simulink model "apollo_longitude"  (R2018a)
settings: Solver=VariableStepAuto  StartTime=0.0  StopTime=200  RelTol=1e-5
undefined symbols (not defined in the file): high_speed_Ki, high_speed_Kp, ref_station, speed_controller_input_limit, station_Kp
settings Model: Creator=cidi-xh  LastModifiedBy=DELL

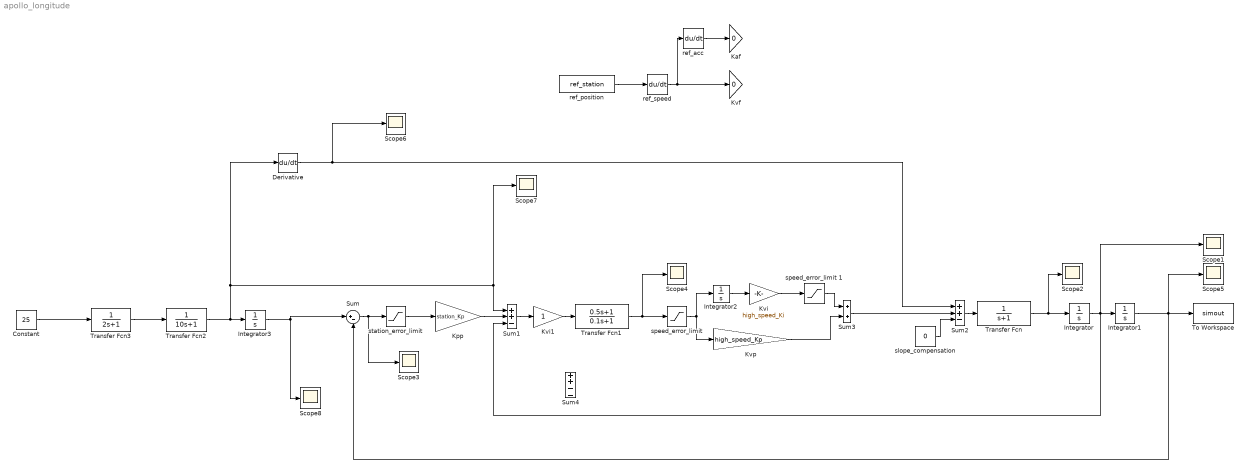
== system apollo_longitude ==
  Constant : Constant  Value=25
  Derivative : Derivative
  Integrator{,1..3} (4 alike) : Integrator
  Kaf : Gain  Gain=0
  Kpp : Gain  Gain=station_Kp
  Kvf : Gain  Gain=0
  Kvi : Gain  Gain=high_speed_Ki
  Kvi1 : Gain
  Kvp : Gain  Gain=high_speed_Kp
  Scope{1..8} (8 alike) : Scope
  Sum : Sum  Inputs=|+-
  Sum1 : Sum  Inputs=++-
  Sum2 : Sum  Inputs=++-
  Sum3 : Sum
  Sum4 : Sum  Inputs=++--
  To Workspace : ToWorkspace  VariableName=simout  SaveFormat=Timeseries  SampleTime=-1
  Transfer Fcn : TransferFcn  Denominator=[1 1]
  Transfer Fcn1 : TransferFcn  Numerator=[0.5 1]  Denominator=[0.1 1]
  Transfer Fcn2 : TransferFcn  Denominator=[10 1]
  Transfer Fcn3 : TransferFcn  Denominator=[2 1]
  "ref_acc " : Derivative
  ref_position : Constant  Value=ref_station
  ref_speed : Derivative
  slope_compensation : Constant  Value=0
  "speed_error_limit " : Saturate  UpperLimit=speed_controller_input_limit  LowerLimit=-speed_controller_input_limit
  speed_error_limit 1 : Saturate  UpperLimit=speed_controller_input_limit  LowerLimit=-speed_controller_input_limit
  "station_error_limit " : Saturate  UpperLimit=speed_controller_input_limit  LowerLimit=-speed_controller_input_limit
  wires:
  Sum/1 -> Scope3/1, "station_error_limit "/1
  "station_error_limit "/1 -> Kpp/1
  Kpp/1 -> Sum1/2
  Transfer Fcn/1 -> Scope2/1, Integrator/1
  Integrator/1 -> Scope1/1, Sum1/3, Integrator1/1
  Integrator1/1 -> Scope5/1, Sum/2, To Workspace/1
  ref_position/1 -> ref_speed/1
  ref_speed/1 -> "ref_acc "/1, Kvf/1
  "ref_acc "/1 -> Kaf/1
  slope_compensation/1 -> Sum2/3
  Sum2/1 -> Transfer Fcn/1
  Sum1/1 -> Kvi1/1
  "speed_error_limit "/1 -> Integrator2/1, Kvp/1
  Integrator2/1 -> Kvi/1
  Kvi/1 -> speed_error_limit 1/1
  Kvp/1 -> Sum3/2
  speed_error_limit 1/1 -> Sum3/1
  Sum3/1 -> Sum2/2
  Kvi1/1 -> Transfer Fcn1/1
  Transfer Fcn1/1 -> Scope4/1, "speed_error_limit "/1
  Constant/1 -> Transfer Fcn3/1
  Transfer Fcn2/1 -> Scope7/1, Sum1/1, Derivative/1, Integrator3/1
  Integrator3/1 -> Scope8/1, Sum/1
  Derivative/1 -> Scope6/1, Sum2/1
  Transfer Fcn3/1 -> Transfer Fcn2/1
